simulink model "optiTruck_Base_Sim_Environment"  (R2016b)
settings: Solver=FixedStepDiscrete  StartTime=0.0  StopTime=100  FixedStep=0.001  RelTol=1e-3  EnableMultiTasking=on
settings Model: Creator=m01wolf  LastModifiedBy=bunver
settings DataIOCC: SaveFormat=StructureWithTime  SaveOutput=off  DSMLogging=off  VisualizeSimOutput=off  SaveTime=off  StateSaveName=Results  SignalLoggingName=Results
settings OptimizationCC: BlockReduction=off  ConditionallyExecuteInputs=off  LifeSpan=inf
settings DebuggingCC: AllowSymbolicDim=off  SFUnexpectedBacktrackingDiag=warning  SFNoUnconditionalDefaultTransitionDiag=warning  SFExecutionAtInitializationDiag=none
settings HardwareCC: ProdBitPerSizeT=32  ProdBitPerPtrDiffT=32  ProdWordSize=32  ProdHWDeviceType=Specified
settings ModelReferenceCC: PropagateSignalLabelsOutOfModel=off
settings GRTTargetCC: TargetLangStandard=C89/C90 (ANSI)
settings ConfigComp: CovMetricSettings=dw  CovHtmlReporting=on  CovSaveCumulativeToWorkspaceVar=on  CovSaveSingleToWorkspaceVar=on  CovExternalEMLEnable=off

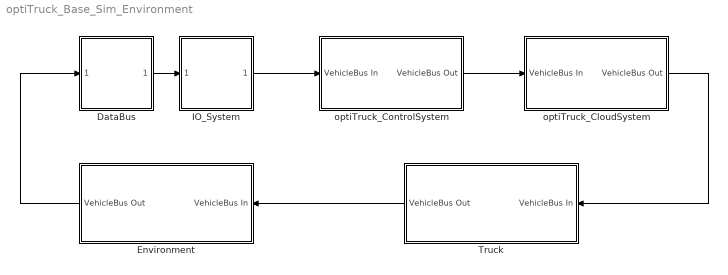
== system optiTruck_Base_Sim_Environment ==
  DataBus : Subsystem
      mask Display: %image('Databus.jpg')
  Environment : Subsystem
      mask Display: %image('Long_Haul_Truck.jpg')
  IO_System : Subsystem
      mask Display: %image('Databus.jpg')
  Truck : Subsystem
      mask Display: %image('Long_Haul_Truck.jpg')
  optiTruck_CloudSystem : Subsystem
      mask Display: %image('optiTruck_Logo.jpg')
  optiTruck_ControlSystem : Subsystem
      mask Display: %image('optiTruck_Logo.jpg')
  wires:
  DataBus/1(VehicleBus Out) -> IO_System/1(VehicleBus In)
  Environment/1(VehicleBus Out) -> DataBus/1(VehicleBus In)
  Truck/1(VehicleBus Out) -> Environment/1(VehicleBus In)
  optiTruck_CloudSystem/1(VehicleBus Out) -> Truck/1(VehicleBus In)
  optiTruck_ControlSystem/1(VehicleBus Out) -> optiTruck_CloudSystem/1(VehicleBus In)
  IO_System/1(VehicleBus Out) -> optiTruck_ControlSystem/1(VehicleBus In)

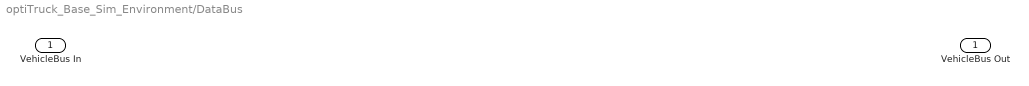
== system optiTruck_Base_Sim_Environment/DataBus ==
  VehicleBus In : Inport
  VehicleBus Out : Outport

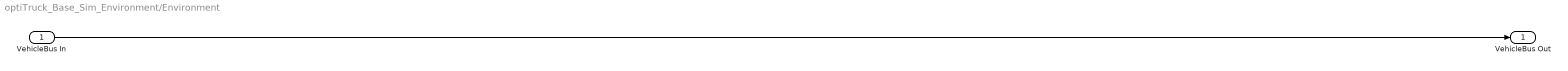
== system optiTruck_Base_Sim_Environment/Environment ==
  VehicleBus In : Inport
  VehicleBus Out : Outport
  wires:
  VehicleBus In/1 -> VehicleBus Out/1

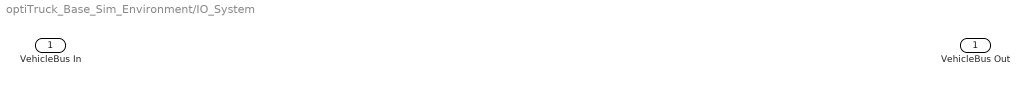
== system optiTruck_Base_Sim_Environment/IO_System ==
  VehicleBus In : Inport
  VehicleBus Out : Outport

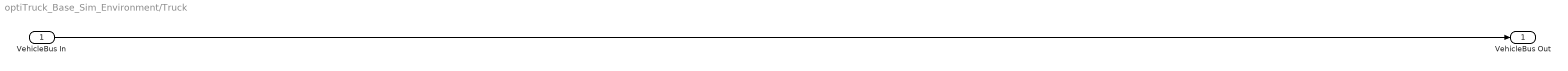
== system optiTruck_Base_Sim_Environment/Truck ==
  VehicleBus In : Inport
  VehicleBus Out : Outport
  wires:
  VehicleBus In/1 -> VehicleBus Out/1

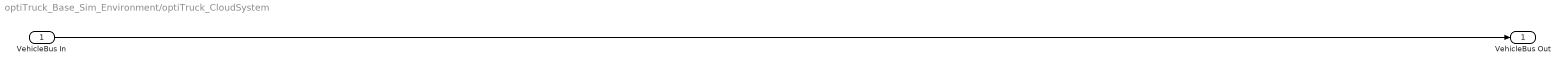
== system optiTruck_Base_Sim_Environment/optiTruck_CloudSystem ==
  VehicleBus In : Inport
  VehicleBus Out : Outport
  wires:
  VehicleBus In/1 -> VehicleBus Out/1

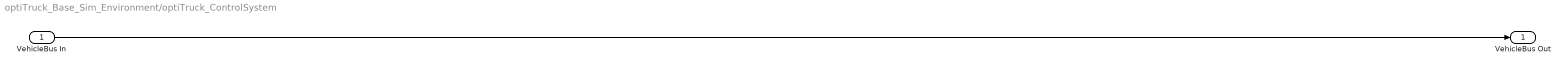
== system optiTruck_Base_Sim_Environment/optiTruck_ControlSystem ==
  VehicleBus In : Inport
  VehicleBus Out : Outport
  wires:
  VehicleBus In/1 -> VehicleBus Out/1
